simulink model "LAB_06_7_NOV_GG_fun"  (R2022b)
settings: Solver=ode4  StartTime=0.0  StopTime=1000  FixedStep=0.01  RelTol=1e-3
values from neighbouring files (symbols this model uses):
  A0 = diag([1 1 1])    [LAB_04_17_OCT_MAT_KIN.m]    (also in LAB_05_24_OCT_MAT_KIN_COSDIR.m; LAB_06.m = A_target_fun(0); core_attitude_test.m = eye(3,3); lab_07_MAT.m)
  I = [Ix 0 0 ... (first row only)    [LAB_03_3_OCT_MAT_EUL_2_VERIFICATION.m]    (also in LAB_03_3_OCT_MAT_EUL_DOUBLESPIN.m = diag([Ix, Iy, Iz]); LAB_03_3_OCT_MAT_EUL_SPINAXIS.m = diag([Ix, Iy, Iz]); LAB_03_3_OCT_MAT_EUL_VECT.m; LAB_04_17_OCT_MAT_KIN.m)
  n = sqrt(n2)    [LAB_06.m]    (also in lab_07_MAT.m)
  om_0 = [om_x0, om_y0, om_z0]    [LAB_03_3_OCT_MAT_EUL.m]    (also in LAB_03_3_OCT_MAT_EUL_2_VERIFICATION.m = [om_x0; om_y0; om_z0]; LAB_03_3_OCT_MAT_EUL_DOUBLESPIN.m = [om_x0; om_y0; om_z0]; LAB_03_3_OCT_MAT_EUL_SPINAXIS.m = [om_x0; om_y0; om_z0]; LAB_03_3_OCT_MAT_EUL_VECT.m = [om_x0; om_y0; om_z0])
  om_target = [0; 0; n]    [LAB_06.m]    (also in lab_07_MAT.m)
libraries: sharedutil x1, matrix_library x1
settings Model: Creator=maria  LastModifiedBy=maria

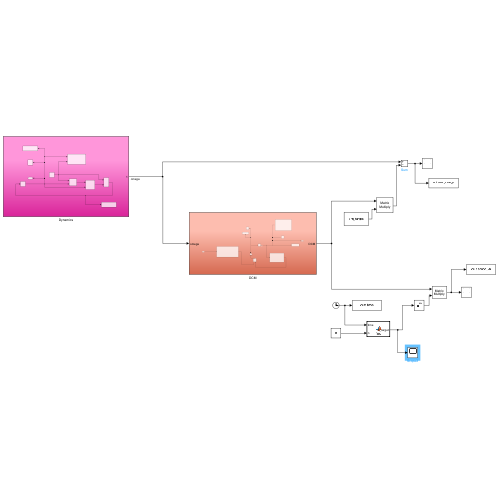
[thumbnail: Simulink's stored preview of the top-level diagram]
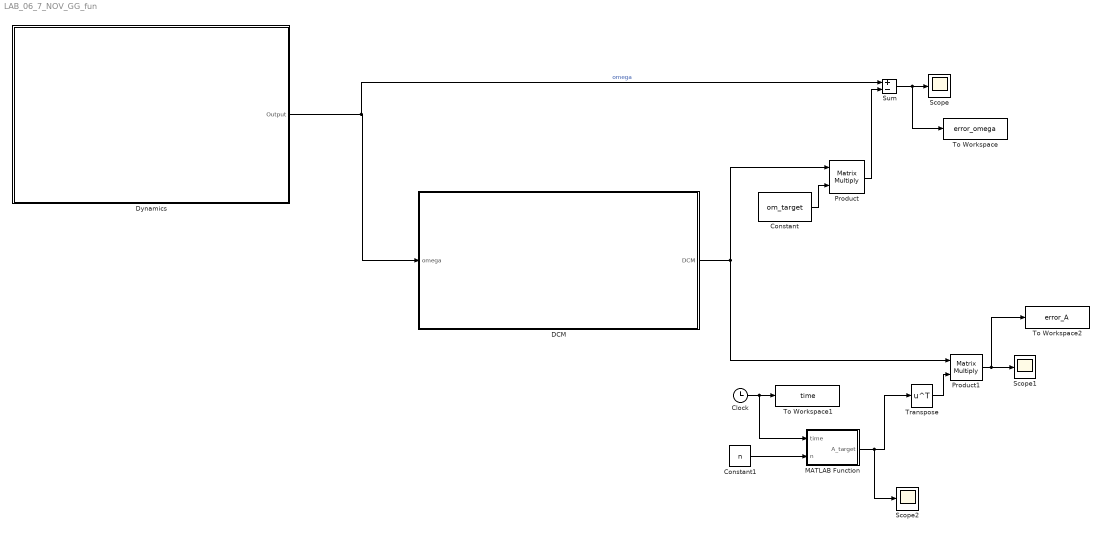
== system LAB_06_7_NOV_GG_fun ==
  Clock : Clock
  Constant : Constant  Value=om_target
  Constant1 : Constant  Value=n
  DCM : Subsystem
  Dynamics : Subsystem
  MATLAB Function : MATLAB Function  TreatAsAtomicUnit=on
  Product : Product  Multiplication=Matrix(*)
  Product1 : Product  Multiplication=Matrix(*)
  Scope : Scope
  Scope1 : Scope
  Scope2 : Scope
  Sum : Sum  Inputs=+-
  To Workspace : ToWorkspace  VariableName=error_omega  SampleTime=-1
  To Workspace1 : ToWorkspace  VariableName=time  SampleTime=-1
  To Workspace2 : ToWorkspace  VariableName=error_A  SampleTime=-1
  Transpose : Math  Operator=transpose
  wires:
  Dynamics/1(Output) -> Sum/1, DCM/1(omega)  "omega"
  DCM/1(DCM) -> Product1/1, Product/1
  Constant/1 -> Product/2
  Product/1 -> Sum/2
  Sum/1 -> To Workspace/1, Scope/1
  Clock/1 -> MATLAB Function/1(time), To Workspace1/1
  MATLAB Function/1(A_target) -> Scope2/1, Transpose/1
  Transpose/1 -> Product1/2
  Product1/1 -> To Workspace2/1, Scope1/1
  Constant1/1 -> MATLAB Function/2(n)

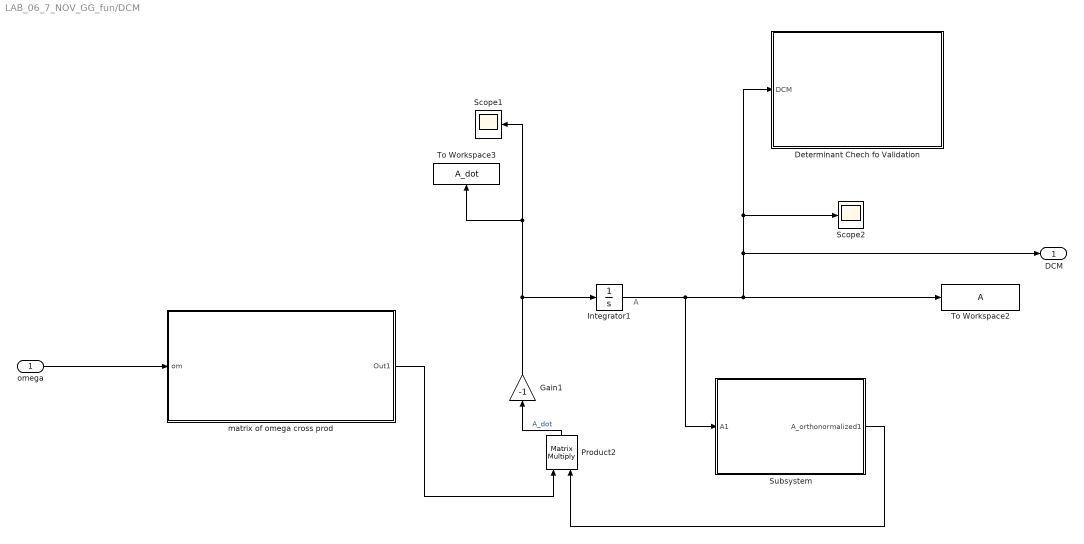
== system LAB_06_7_NOV_GG_fun/DCM ==
  note: A
  omega : Inport
  Determinant Chech fo Validation : Subsystem
  Gain1 : Gain  Gain=-1
  Integrator1 : Integrator  InitialCondition=A0
  Product2 : Product  Multiplication=Matrix(*)
  Scope1 : Scope
  Scope2 : Scope
  Subsystem : Subsystem
  To Workspace2 : ToWorkspace  VariableName=A  SampleTime=-1
  To Workspace3 : ToWorkspace  VariableName=A_dot  SampleTime=-1
  matrix of omega cross prod : Subsystem
  DCM : Outport
  wires:
  Integrator1/1 -> Subsystem/1(A1), Scope2/1, Determinant Chech fo Validation/1(DCM), DCM/1, To Workspace2/1
  matrix of omega cross prod/1(Out1) -> Product2/1
  Product2/1 -> Gain1/1  "A_dot"
  omega/1 -> matrix of omega cross prod/1(om)
  Gain1/1 -> Integrator1/1, To Workspace3/1, Scope1/1
  Subsystem/1(A_orthonormalized1) -> Product2/2

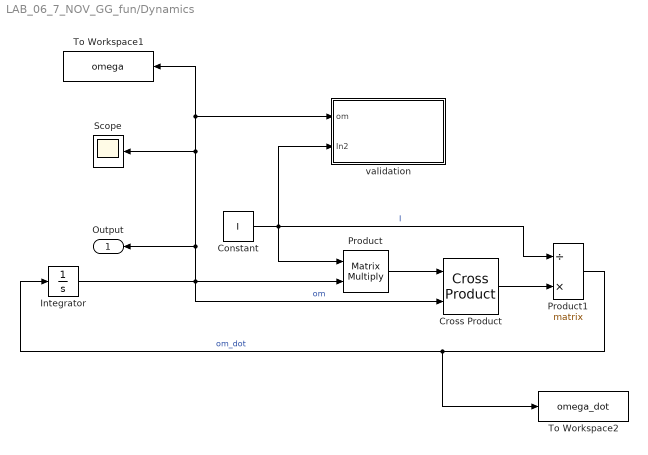
== system LAB_06_7_NOV_GG_fun/Dynamics ==
  Constant : Constant  Value=I
  Cross Product : matrix_library/Cross Product
  Integrator : Integrator  InitialCondition=om_0
  Product : Product  Multiplication=Matrix(*)
  Product1 : Product  Inputs=/*  Multiplication=Matrix(*)
  Scope : Scope
  To Workspace1 : ToWorkspace  VariableName=omega  SampleTime=-1
  To Workspace2 : ToWorkspace  VariableName=omega_dot  SampleTime=-1
  validation : Subsystem
  Output : Outport
  wires:
  Product1/1 -> To Workspace2/1, Integrator/1  "om_dot"
  Integrator/1 -> Product/2, Cross Product/2, validation/1(om), To Workspace1/1, Scope/1, Output/1  "om"
  Cross Product/1 -> Product1/2
  Constant/1 -> Product1/1, Product/1, validation/2(In2)  "I"
  Product/1 -> Cross Product/1

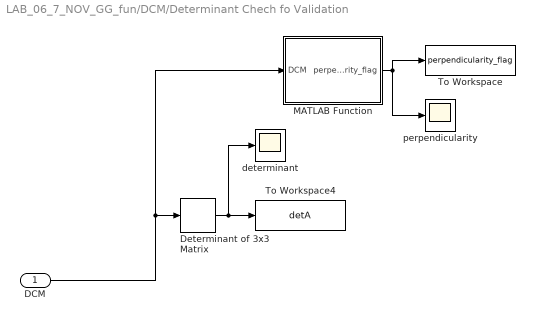
== system LAB_06_7_NOV_GG_fun/DCM/Determinant Chech fo Validation ==
  DCM : Inport
  Determinant of 3x3 Matrix : sharedutil/Determinant of 3x3 Matrix  aMode=aMode
      settings: LibrarySourceBlock=|
      | aerolibutil/Determinant of
      | 3x3 Matrix
  MATLAB Function : MATLAB Function  TreatAsAtomicUnit=on
  To Workspace : ToWorkspace  VariableName=perpendicularity_flag  SampleTime=-1
  To Workspace4 : ToWorkspace  VariableName=detA  SampleTime=-1
  determinant : Scope
  perpendicularity : Scope
  wires:
  Determinant of 3x3 Matrix/1 -> determinant/1, To Workspace4/1
  DCM/1 -> MATLAB Function/1(DCM), Determinant of 3x3 Matrix/1
  MATLAB Function/1(perpendicularity_flag) -> To Workspace/1, perpendicularity/1

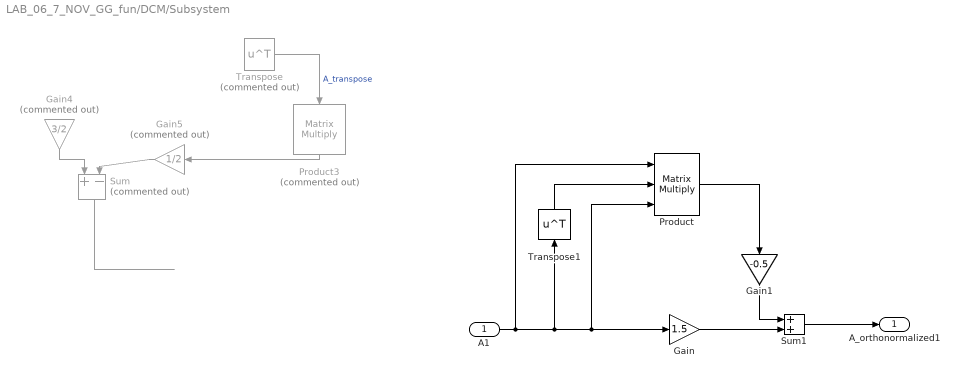
== system LAB_06_7_NOV_GG_fun/DCM/Subsystem ==
  A1 : Inport
  Gain : Gain  Gain=1.5
  Gain1 : Gain  Gain=-0.5
  Gain4 : Gain  Commented=on  Gain=3/2
  Gain5 : Gain  Commented=on  Gain=1/2
  Product : Product  Inputs=3  Multiplication=Matrix(*)
  Product3 : Product  Commented=on  Inputs=3  Multiplication=Matrix(*)
  Sum : Sum  Commented=on  Inputs=+-
  Sum1 : Sum
  Transpose : Math  Commented=on  Operator=transpose
  Transpose1 : Math  Operator=transpose
  A_orthonormalized1 : Outport
  wires:
  Sum/1 -> ?
  Gain5/1 -> Sum/2
  Product3/1 -> Gain5/1
  Transpose/1 -> Product3/2  "A_transpose"
  Gain4/1 -> Sum/1
  A1/1 -> Product/1, Transpose1/1, Product/3, Gain/1
  Gain/1 -> Sum1/2
  Sum1/1 -> A_orthonormalized1/1
  Gain1/1 -> Sum1/1
  Product/1 -> Gain1/1
  Transpose1/1 -> Product/2

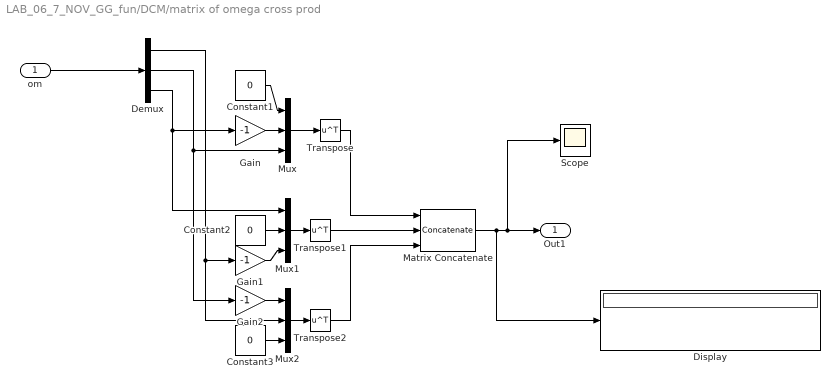
== system LAB_06_7_NOV_GG_fun/DCM/matrix of omega cross prod ==
  om : Inport
  Constant1 : Constant  Value=0
  Constant2 : Constant  Value=0
  Constant3 : Constant  Value=0
  Demux : Demux  Outputs=3
  Display : Display
  Gain : Gain  Gain=-1
  Gain1 : Gain  Gain=-1
  Gain2 : Gain  Gain=-1
  Matrix Concatenate : Concatenate  NumInputs=3  Mode=Multidimensional array
  Mux : Mux  Inputs=3
  Mux1 : Mux  Inputs=3
  Mux2 : Mux  Inputs=3
  Scope : Scope
  Transpose : Math  Operator=transpose
  Transpose1 : Math  Operator=transpose
  Transpose2 : Math  Operator=transpose
  Out1 : Outport
  wires:
  Matrix Concatenate/1 -> Display/1, Scope/1, Out1/1
  Demux/1 -> Gain1/1, Mux2/2
  Mux1/1 -> Transpose1/1
  Constant3/1 -> Mux2/3
  Gain/1 -> Mux/2
  Gain2/1 -> Mux2/1
  Constant1/1 -> Mux/1
  Demux/3 -> Gain/1, Mux1/1
  Demux/2 -> Mux/3, Gain2/1
  Mux/1 -> Transpose/1
  Gain1/1 -> Mux1/3
  Mux2/1 -> Transpose2/1
  Constant2/1 -> Mux1/2
  om/1 -> Demux/1
  Transpose/1 -> Matrix Concatenate/1
  Transpose1/1 -> Matrix Concatenate/2
  Transpose2/1 -> Matrix Concatenate/3

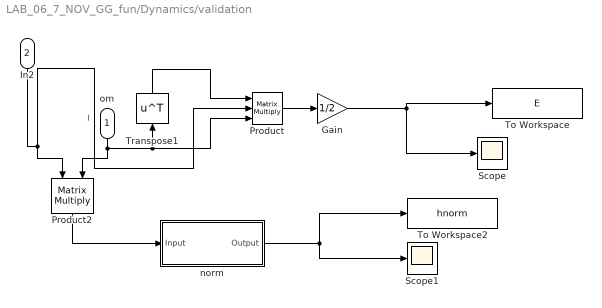
== system LAB_06_7_NOV_GG_fun/Dynamics/validation ==
  om : Inport
  In2 : Inport  Port=2
  Gain : Gain  Gain=1/2
  Product : Product  Inputs=3  Multiplication=Matrix(*)
  Product2 : Product  Multiplication=Matrix(*)
  Scope : Scope
  Scope1 : Scope
  To Workspace : ToWorkspace  VariableName=E  SampleTime=-1
  To Workspace2 : ToWorkspace  VariableName=hnorm  SampleTime=-1
  Transpose1 : Math  Operator=transpose
  norm : Subsystem
  wires:
  Product2/1 -> norm/1(Input)
  norm/1(Output) -> To Workspace2/1, Scope1/1
  om/1 -> Transpose1/1, Product/3, Product2/2
  In2/1 -> Product/2, Product2/1  "I"
  Transpose1/1 -> Product/1
  Product/1 -> Gain/1
  Gain/1 -> Scope/1, To Workspace/1

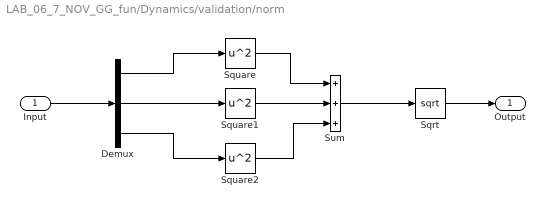
== system LAB_06_7_NOV_GG_fun/Dynamics/validation/norm ==
  Input : Inport
  Demux : Demux  Outputs=3
  Sqrt : Sqrt
  Square : Math  Operator=square
  Square1 : Math  Operator=square
  Square2 : Math  Operator=square
  Sum : Sum  Inputs=+++
  Output : Outport
  wires:
  Square/1 -> Sum/1
  Square1/1 -> Sum/2
  Square2/1 -> Sum/3
  Sum/1 -> Sqrt/1
  Input/1 -> Demux/1
  Sqrt/1 -> Output/1
  Demux/1 -> Square/1
  Demux/2 -> Square1/1
  Demux/3 -> Square2/1

== matlab function LAB_06_7_NOV_GG_fun/DCM/Determinant Chech fo Validation/MATLAB Function ==
  data: DCM input; perpendicularity_flag output
function perpendicularity_flag = fcn(DCM)


perpendicularity_flag =zeros(3,1);

    x   = DCM(1,:);
    y   = DCM(2,:);
    z   = DCM(3,:);

    perpendicularity_flag(1)=dot(x,y);
    perpendicularity_flag(2)=dot(x,z);
    perpendicularity_flag(3)=dot(z,y);

end

== matlab function LAB_06_7_NOV_GG_fun/MATLAB Function ==
  data: time input; A_target output; n input
function A_target = fnc(time, n)

t = time;
A_target = [cos(n*t), sin(n*t), 0;
            -sin(n*t), cos(n*t), 0;
             0, 0, 1];
